simulink model "booster_observer"  (R2024b)
settings: Solver=VariableStepAuto  StartTime=0.0  StopTime=Tfin_obs  RelTol=1e-3
values from neighbouring files (symbols this model uses):
  a = pi*r^2    (= 78.5398163397)    [script_project.m]
  Aobs = A-L*C    [script_project.m]
  Bobs = [B L]    [script_project.m]
  Cd = 1.2    [script_project.m]
  Cobs = eye(4)    [script_project.m]
  Dobs = zeros(4, 5)    [script_project.m]
  g = 9.81    [script_project.m]
  h = 70    [script_project.m]
  J = (1/12)*m*(b^2 + h^2)    (= 208333333.333)    [script_project.m]
  m = 500000    [script_project.m]
  rho = 1.225    [script_project.m]
  u0 = [u1eq u2eq u3eq]'    [script_project.m]
  z0_obs = z0 + dz0_obs    [script_project.m]
undefined symbols (not defined in the file or in its folder): A, B, C
settings Model: Creator=martinhaugen  LastModifiedBy=martinhaugen

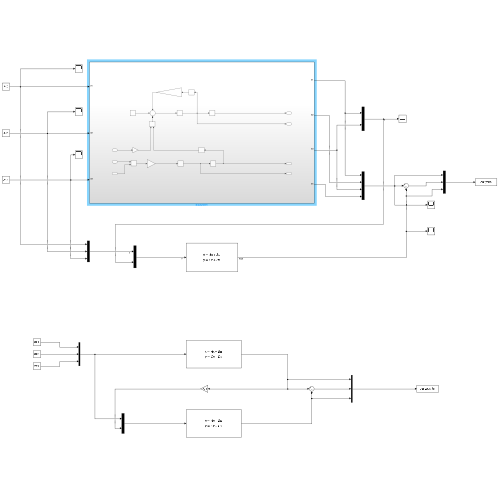
[thumbnail: Simulink's stored preview of the top-level diagram]
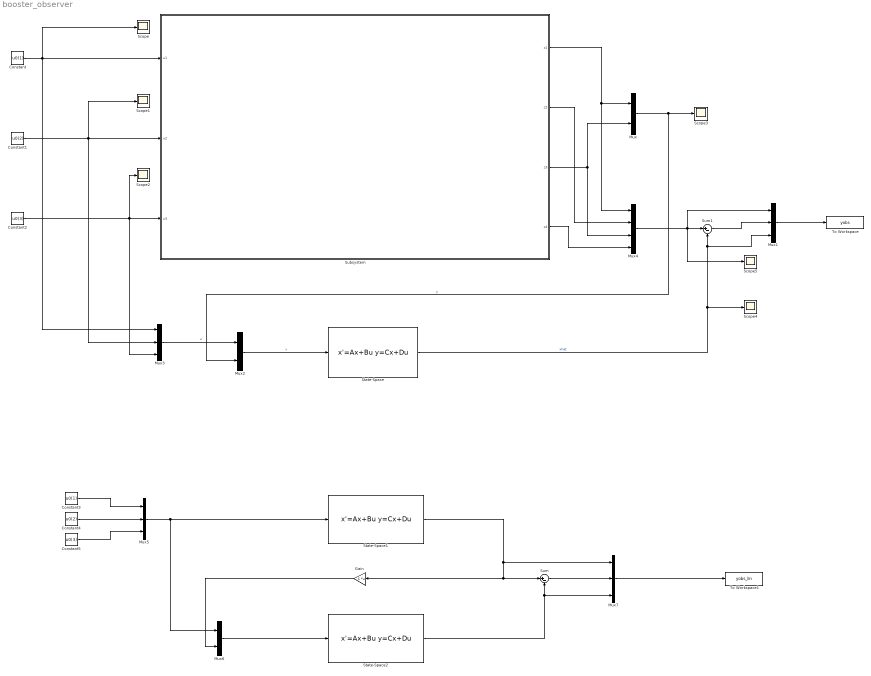
== system booster_observer ==
  Constant : Constant  Value=u0(1)
  Constant1 : Constant  Value=u0(2)
  Constant2 : Constant  Value=u0(3)
  Constant3 : Constant  Value=u0(1)
  Constant4 : Constant  Value=u0(2)
  Constant5 : Constant  Value=u0(3)
  Gain : Gain  Gain=C  Multiplication=Matrix(K*u)
  Mux : Mux  Inputs=2
  Mux{1,3,5,7} (4 alike) : Mux  Inputs=3
  Mux2 : Mux  Inputs=2
  Mux4 : Mux
  Mux6 : Mux  Inputs=2
  Scope{,1..5} (6 alike) : Scope
  State-Space : StateSpace  A=Aobs  B=Bobs  C=Cobs  D=Dobs  InitialCondition=z0_obs
  State-Space1 : StateSpace  A=A  B=B  C=eye(4)  D=zeros(4,3)  InitialCondition=z0_obs
  State-Space2 : StateSpace  A=Aobs  B=Bobs  C=Cobs  D=Dobs  InitialCondition=z0_obs
  Subsystem : Subsystem
  Sum : Sum  Inputs=|+-
  Sum1 : Sum  Inputs=|+-
  To Workspace : ToWorkspace  VariableName=yobs  SaveFormat=Timeseries  SampleTime=-1
  To Workspace1 : ToWorkspace  VariableName=yobs_lin  SaveFormat=Timeseries  SampleTime=-1
  wires:
  Constant2/1 -> Scope2/1, Subsystem/3(u3), Mux3/3
  Constant/1 -> Mux3/1, Subsystem/1(u1), Scope/1
  Subsystem/3(z3) -> Mux4/3, Mux/2
  Constant1/1 -> Mux3/2, Subsystem/2(u2), Scope1/1
  Subsystem/1(z1) -> Mux/1, Mux4/1
  Mux1/1 -> To Workspace/1
  Mux/1 -> Scope3/1, Mux2/2  "y"
  Mux2/1 -> State-Space/1  "v"
  State-Space/1 -> Scope4/1, Sum1/2, Mux1/3  "xhat"
  Mux3/1 -> Mux2/1  "u"
  Subsystem/2(z2) -> Mux4/2
  Subsystem/4(z4) -> Mux4/4
  Mux4/1 -> Sum1/1, Mux1/1, Scope5/1
  Sum1/1 -> Mux1/2
  Constant4/1 -> Mux5/2
  Constant3/1 -> Mux5/1
  Constant5/1 -> Mux5/3
  Mux5/1 -> State-Space1/1, Mux6/1
  State-Space1/1 -> Gain/1, Sum/1, Mux7/1
  Mux6/1 -> State-Space2/1
  State-Space2/1 -> Sum/2, Mux7/3
  Sum/1 -> Mux7/2
  Mux7/1 -> To Workspace1/1
  Gain/1 -> Mux6/2

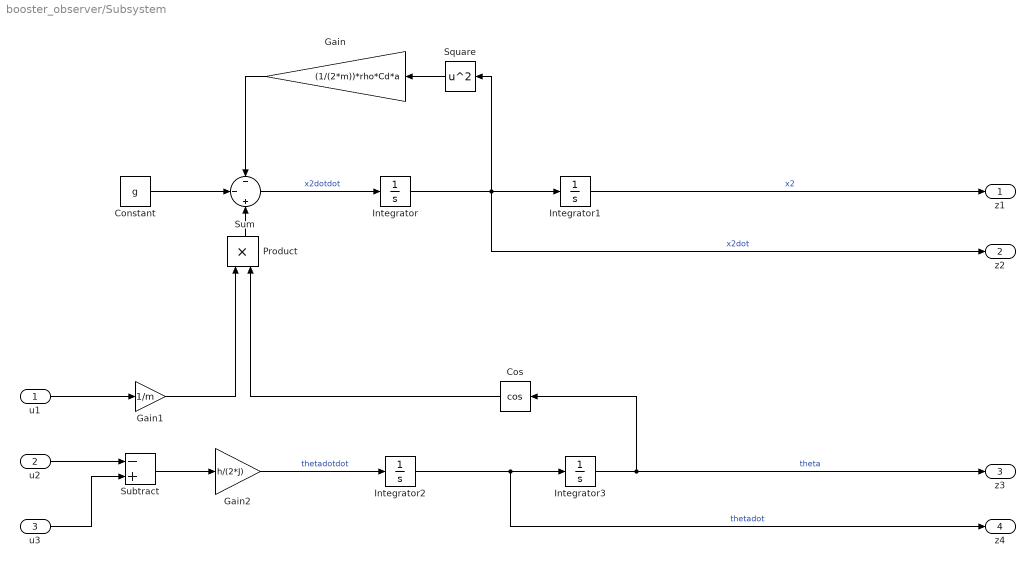
== system booster_observer/Subsystem ==
  u1 : Inport
  u2 : Inport  Port=2
  u3 : Inport  Port=3
  Constant : Constant  Value=g
  Cos : Trigonometry  Operator=cos
  Gain : Gain  Gain=(1/(2*m))*rho*Cd*a
  Gain1 : Gain  Gain=1/m
  Gain2 : Gain  Gain=h/(2*J)
  Integrator : Integrator  InitialCondition=z0_obs(2)  ContinuousStateAttributes='z2'
  Integrator1 : Integrator  InitialCondition=z0_obs(1)  ContinuousStateAttributes='z1'
  Integrator2 : Integrator  InitialCondition=z0_obs(4)  ContinuousStateAttributes='z4'
  Integrator3 : Integrator  InitialCondition=z0_obs(3)  ContinuousStateAttributes='z3'
  Product : Product
  Square : Math  Operator=square
  Subtract : Sum  Inputs=-+
  Sum : Sum  Inputs=-|-|+
  z1 : Outport
  z2 : Outport  Port=2
  z3 : Outport  Port=3
  z4 : Outport  Port=4
  wires:
  u2/1 -> Subtract/1
  Constant/1 -> Sum/2
  Square/1 -> Gain/1
  Product/1 -> Sum/3
  Subtract/1 -> Gain2/1
  Integrator/1 -> z2/1, Integrator1/1, Square/1  "x2dot"
  Gain2/1 -> Integrator2/1  "thetadotdot"
  Cos/1 -> Product/2
  u3/1 -> Subtract/2
  Integrator2/1 -> z4/1, Integrator3/1  "thetadot"
  u1/1 -> Gain1/1
  Gain/1 -> Sum/1
  Sum/1 -> Integrator/1  "x2dotdot"
  Gain1/1 -> Product/1
  Integrator3/1 -> z3/1, Cos/1  "theta"
  Integrator1/1 -> z1/1  "x2"
